simulink model "observer_reduced"  (R2023b)
settings: Solver=VariableStepAuto  StartTime=0.0  StopTime=50.0  RelTol=1e-3
values from neighbouring files (symbols this model uses):
  A = [ -8.8487+(a-b)/5,           -0.0399,                     -5.55+(c+d)/10,               3.5846 ... (first row only)    [EE5101_Q1 copy.m]    (also in EE5101_Q1.m; Q3.m; Q3_reduced_order.m; Q6.m)
  B = [0.0564+b/(10+c),                       0.0319 ... (first row only)    [EE5101_Q1 copy.m]    (also in EE5101_Q1.m; Q3.m; Q3_reduced_order.m; Q6.m)
  C = [-3.2988,              -2.1932+(10*c+d)/(100+5*a),  0.037,      -0.0109 ... (first row only)    [EE5101_Q1 copy.m]    (also in EE5101_Q1.m; Q3.m; Q3_reduced_order.m; Q6.m)
  D = [-5 0 ... (first row only)    [Q3_reduced_order.m]
  E = double(T*B)    [Q3_reduced_order.m]
  G = [g1 0 ... (first row only)    [Q3_reduced_order.m]
  K_LQR = lqr(A, B, Q1, R)    [Q3.m]    (also in Q6.m = inv(R)*B'*P -inv(R)*[])
  T_new = inv([C; T])    [Q3_reduced_order.m]
settings Model: Creator=wyton  LastModifiedBy=shipingguo
settings SolverCC: AlgebraicLoopSolver=TrustRegion
settings OptimizationCC: ReuseModelBlockBuffer=off
settings DebuggingCC: UnconnectedInputMsg=warning  UnconnectedOutputMsg=warning  UnconnectedLineMsg=warning
settings ModelReferenceCC: EnableRefExpFcnMdlSchedulingChecks=on
settings RTWCC: DLArmComputeVersion=19.05

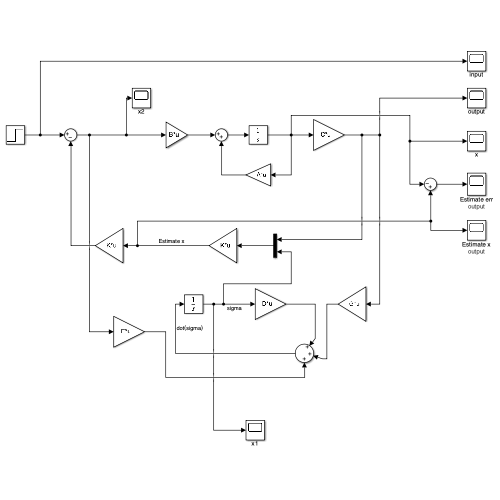
[thumbnail: Simulink's stored preview of the top-level diagram]
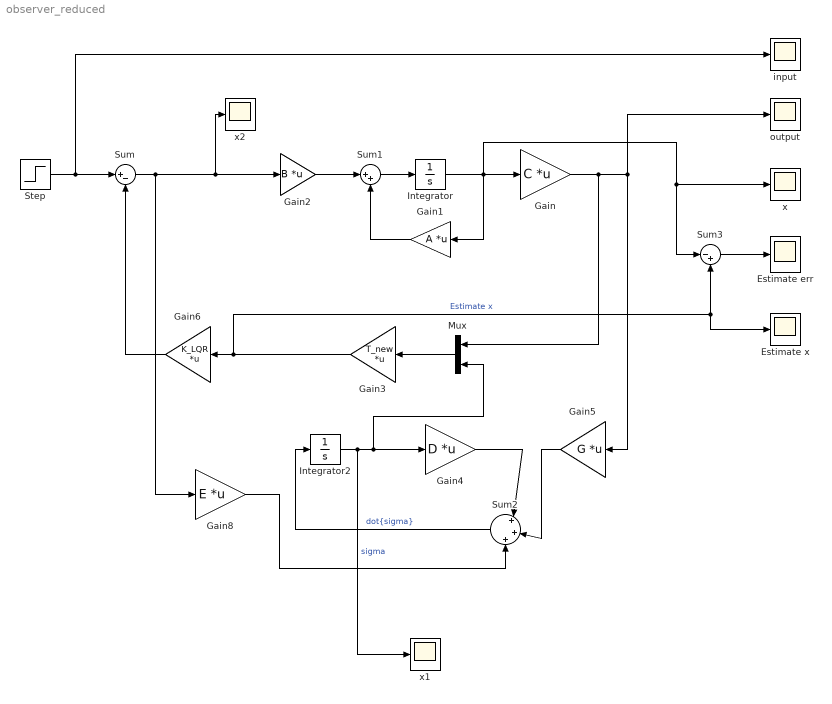
== system observer_reduced ==
  Estimate err : Scope
      settings: AttributesFormatString=output
  Estimate x : Scope
      settings: AttributesFormatString=output
  Gain : Gain  Gain=C  Multiplication=Matrix(K*u)
  Gain1 : Gain  Gain=A  Multiplication=Matrix(K*u)
  Gain2 : Gain  Tag=B  Gain=B  Multiplication=Matrix(K*u)
  Gain3 : Gain  Gain=T_new  Multiplication=Matrix(K*u)
  Gain4 : Gain  Gain=D  Multiplication=Matrix(K*u)
  Gain5 : Gain  Gain=G  Multiplication=Matrix(K*u)
  Gain6 : Gain  Gain=K_LQR  Multiplication=Matrix(K*u)
  Gain8 : Gain  Gain=E  Multiplication=Matrix(K*u)
  Integrator : Integrator  InitialCondition=[0.5 -0.1 0.1 -0.8]
  Integrator2 : Integrator  InitialCondition=[0 0]
  Mux : Mux  Inputs=2
  Step : Step  Time=0  Before=[0,0]  After=[0;0]  SampleTime=0
  Sum : Sum  Inputs=|+-
  Sum1 : Sum  Inputs=|++
  Sum2 : Sum  Inputs=|+|+|+
  Sum3 : Sum  Inputs=|-+
  input : Scope
  output : Scope
  x : Scope
  x1 : Scope
  x2 : Scope
  wires:
  Step/1 -> Sum/1, input/1
  Sum1/1 -> Integrator/1
  Gain2/1 -> Sum1/1
  Gain1/1 -> Sum1/2
  Integrator/1 -> Gain1/1, Sum3/1, x/1, Gain/1
  Gain/1 -> Mux/1, output/1, Gain5/1
  Integrator2/1 -> x1/1, Mux/2, Gain4/1  "sigma"
  Gain4/1 -> Sum2/1
  Gain5/1 -> Sum2/2
  Sum2/1 -> Integrator2/1  "dot{sigma}"
  Mux/1 -> Gain3/1
  Gain3/1 -> Gain6/1, Sum3/2, Estimate x/1  "Estimate x"
  Sum3/1 -> Estimate err/1
  Gain8/1 -> Sum2/3
  Sum/1 -> x2/1, Gain2/1, Gain8/1
  Gain6/1 -> Sum/2
